simulink model "rangefinder"  (Simulink 7.0)
settings: Solver=ode14x  StartTime=0.0  StopTime=30  FixedStep=0.001  RelTol=1e-3
undefined symbols (not defined in the file): Model_626, Sensoray
libraries: dspsigops x4, dspsnks4 x4, rtwinlib x2, simulink x1
settings Model: Creator=Student  LastModifiedBy=Student  SimulationMode=external  ExtModeTrigDuration=60000
settings DataIOCC: MaxDataPoints=60000
settings HardwareCC: ProdHWDeviceType=Generic->32-bit Real-Time Simulator  TargetHWDeviceType=32-bit Generic  ProdEqTarget=off
settings RTWCC: SystemTargetFile=rtwin.tlc  TemplateMakefile=rtwin.tmf  Description=Real-Time Windows Target  ProcessScript=rtwin_make_rtw_hook
settings RTWinTargetCC: GenFloatMathFcnCalls=ANSI_C  ModelReferenceCompliant=off  CompOptLevelCompliant=off  PortableWordSizes=off  CCOptimize=on

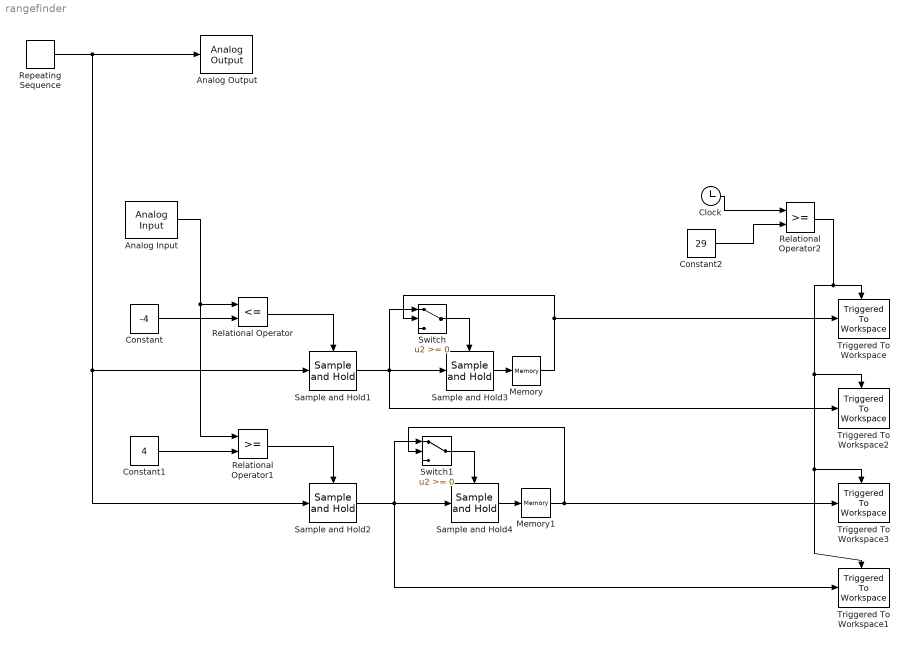
== system rangefinder ==
  Analog Input : rtwinlib/Analog Input  SampleTime=-1  DrvName=Sensoray/Model_626  DrvAddress=4294967295  DrvOptions=zeros(1,0)  Channels=1  RangeMode=1  VoltRange=1  DataType=1
      settings: AttributesFormatString=Sensoray\nModel 626 [auto]
  Analog Output : rtwinlib/Analog Output  SampleTime=-1  DrvName=Sensoray/Model_626  DrvAddress=4294967295  DrvOptions=zeros(1,0)  Channels=1  RangeMode=1  VoltRange=1  InitialValue=0  FinalValue=0
      settings: AttributesFormatString=Sensoray\nModel 626 [auto]
  Clock : Clock
      settings: Decimation=10
  Constant : Constant  Value=-4  OutDataType=sfix(16)  OutScaling=2^0
  Constant1 : Constant  Value=4  OutDataType=sfix(16)  OutScaling=2^0
  Constant2 : Constant  Value=29  OutDataType=sfix(16)  OutScaling=2^0
  Memory : Memory
  Memory1 : Memory
  Relational Operator : RelationalOperator  Operator=<=  LogicOutDataTypeMode=boolean
  Relational Operator1 : RelationalOperator  LogicOutDataTypeMode=boolean
  Relational Operator2 : RelationalOperator  LogicOutDataTypeMode=boolean
  Repeating Sequence : simulink/Sources/Repeating Sequence  SystemSampleTime=-1  rep_seq_t=[0 30]  rep_seq_y=[0.2 4]
  Sample and Hold1 : dspsigops/Sample and Hold  SystemSampleTime=-1  trig=Either edge  initCond=0  latchinput=off
  Sample and Hold2 : dspsigops/Sample and Hold  SystemSampleTime=-1  trig=Either edge  initCond=0  latchinput=off
  Sample and Hold3 : dspsigops/Sample and Hold  SystemSampleTime=-1  trig=Rising edge  initCond=0  latchinput=off
  Sample and Hold4 : dspsigops/Sample and Hold  SystemSampleTime=-1  trig=Rising edge  initCond=0  latchinput=off
  Switch : Switch  OutDataType=sfix(16)  OutScaling=2^0
  Switch1 : Switch  OutDataType=sfix(16)  OutScaling=2^0
  Triggered To Workspace : dspsnks4/Triggered To Workspace  SystemSampleTime=-1  TriggerType=Rising edge  VariableName=SaturationMin  Buffer=1
      settings: FixptAsFi=off
  Triggered To Workspace1 : dspsnks4/Triggered To Workspace  SystemSampleTime=-1  TriggerType=Rising edge  VariableName=SaturationMax  Buffer=1
      settings: FixptAsFi=off
  Triggered To Workspace2 : dspsnks4/Triggered To Workspace  SystemSampleTime=-1  TriggerType=Rising edge  VariableName=DeadMin  Buffer=1
      settings: FixptAsFi=off
  Triggered To Workspace3 : dspsnks4/Triggered To Workspace  SystemSampleTime=-1  TriggerType=Rising edge  VariableName=DeadMax  Buffer=1
      settings: FixptAsFi=off
  wires:
  Analog Input/1 -> Relational Operator/1, Relational Operator1/1
  Repeating Sequence/1 -> Sample and Hold1/1, Sample and Hold2/1, Analog Output/1
  Constant/1 -> Relational Operator/2
  Relational Operator/1 -> Sample and Hold1/Trigger
  Constant1/1 -> Relational Operator1/2
  Relational Operator1/1 -> Sample and Hold2/Trigger
  Switch/1 -> Sample and Hold3/Trigger
  Sample and Hold1/1 -> Sample and Hold3/1, Switch/1, Triggered To Workspace2/1
  Sample and Hold3/1 -> Memory/1
  Switch1/1 -> Sample and Hold4/Trigger
  Sample and Hold2/1 -> Switch1/1, Sample and Hold4/1, Triggered To Workspace1/1
  Sample and Hold4/1 -> Memory1/1
  Memory1/1 -> Switch1/2, Triggered To Workspace3/1
  Memory/1 -> Switch/2, Triggered To Workspace/1
  Clock/1 -> Relational Operator2/1
  Constant2/1 -> Relational Operator2/2
  Relational Operator2/1 -> Triggered To Workspace/Trigger, Triggered To Workspace2/Trigger, Triggered To Workspace3/Trigger, Triggered To Workspace1/Trigger
